simulink model "EPRModel_doublePulseStimulusCodeOffset"  (R2022a)
settings: Solver=ode5  StartTime=0.0  StopTime=inf  RelTol=1e-3
InitFcn:
  | eprecorder_mdl_init_callback();
StopFcn:
  | eprecorder_mdl_stop_callback;
undefined symbols (not defined in the file or in its folder): EPR, eprecorder_online_on_triggered, eprecorder_online_on_viewer_triggered
libraries: simulink x2, sldrtlib x1
settings Model: Creator=Neurolab  LastModifiedBy=bo11r
settings SolverCC: AlgebraicLoopSolver=TrustRegion
settings DebuggingCC: UnconnectedInputMsg=warning  UnconnectedOutputMsg=warning  UnconnectedLineMsg=warning  SFMachineParentedDataDiag=warning
settings RTWCC: Description=Simulink Desktop Real-Time  SystemTargetFile=sldrt.tlc  TemplateMakefile=sldrt.tmf  RTWCompilerOptimization=on  DLArmComputeVersion=19.05
settings CodeAppCC: MaxIdLength=95
settings SimulinkDesktopRealTimeCC: TargetPreCompLibLocation=C:\Program Files\MATLAB\R2020b\toolbox\sldrt\lib\win64

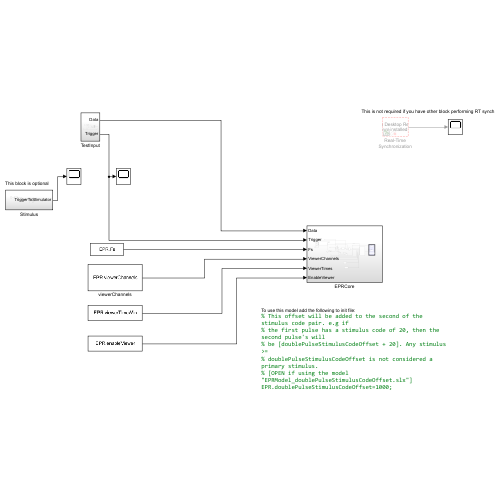
[thumbnail: Simulink's stored preview of the top-level diagram]
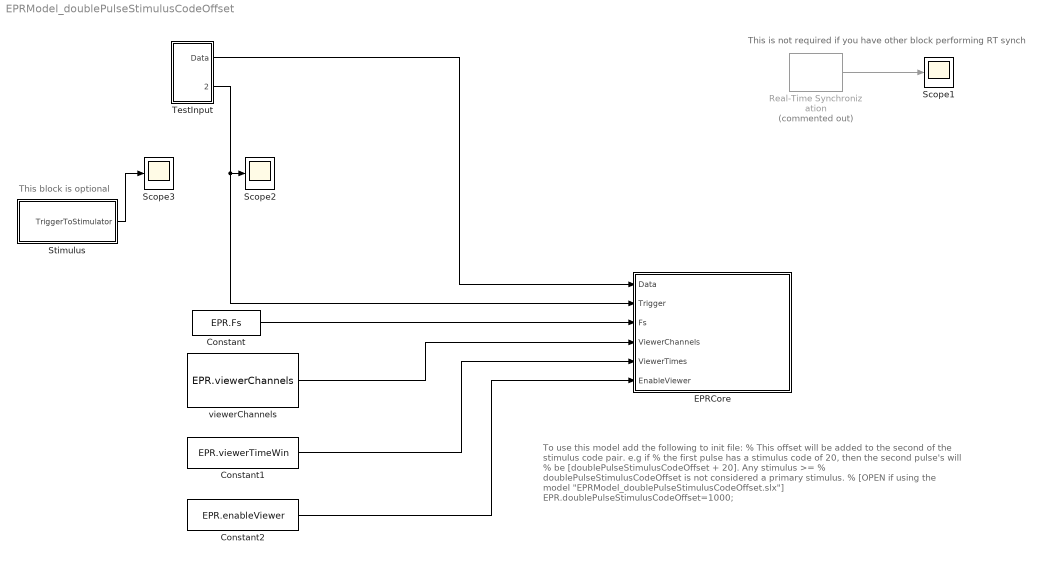
== system EPRModel_doublePulseStimulusCodeOffset ==
  note: To use this model add the following to init file:
      | % This offset will be added to the second of the stimulus code pair. e.g if
      | % the first pulse has a stimulus code of 20, then the second pulse's will
      | % be [doublePulseStimulusCodeOffset + 20]. Any stimulus >=
      | % doublePulseStimulusCodeOffset is not considered a primary stimulus.
      | % [OPEN if using the model "EPRModel_doublePulseStimulusCodeOffset.slx"]
      | EPR.doublePulseStimulusCodeOffset=1000;
  note: This block is optional
  note: This is not required if you have other block performing RT synch
  Constant : Constant  Value=EPR.Fs
  Constant1 : Constant  Value=EPR.viewerTimeWin
  Constant2 : Constant  Value=EPR.enableViewer
  EPRCore : Subsystem
  Real-Time Synchronization : sldrtlib/Real-Time Synchronization  Commented=on  SampleTime=1/EPR.Fs  MaxMissedTicks=1000  ShowMissedTicks=on  YieldWhenWaiting=off
  Scope1 : Scope
  Scope2 : Scope
  Scope3 : Scope
  Stimulus : Subsystem
  TestInput : Subsystem
  viewerChannels : Constant  Value=EPR.viewerChannels  mask(Creates axes for plottint EP){}
      mask init:
      | %{
      |  p=[403   246   560   420]
      |  u='pixels'
      | if(length(findobj('tag','EMG000')))
      |      h=figure(findobj('tag','EMG000'));
      |      p=get(h,'position');
      |      u=get(h,'units');
      |      close(h);
      | end
      |      figure1 = figure('numbertitle','off','name','EP','tag','EMG000');
      |      set(figure1,'units',u);
      |      set(figure1,'position',p);
      |      % Create axes
      |      MYEP.axes(1)=subplot(3,1,1);
      |       title('Channels 1 avg')
      |       box(MYEP.axes(1),'on');
      |       hold(MYEP.axes(1),'all');
      | 
      |      MYEP.axes(2)=subplot(3,1,2);
      |       title('Channels 2 avg')
      |       box(MYEP.axes(2),'on');
      |       hold(MYEP.axes(2),'all');
      | 
      |      MYEP.axes(3)=subplot(3,1,3);
      |      title('Channels 3 avg')
      |      xlabel('1 sec Samples since stimulus onset')
      |      ylabel('Avg amplitude (micro volts)')
      |      box(MYEP.axes(3),'on');
      |      hold(MYEP.axes(3),'all');
      | 
      | %}
  wires:
  viewerChannels/1 -> EPRCore/4(ViewerChannels)
  Constant/1 -> EPRCore/3(Fs)
  Constant1/1 -> EPRCore/5(ViewerTimes)
  Constant2/1 -> EPRCore/6(EnableViewer)
  Real-Time Synchronization/1 -> Scope1/1
  TestInput/1(Data) -> EPRCore/1(Data)
  TestInput/2(Trigger) -> EPRCore/2(Trigger), Scope2/1
  Stimulus/1(TriggerToStimulator) -> Scope3/1

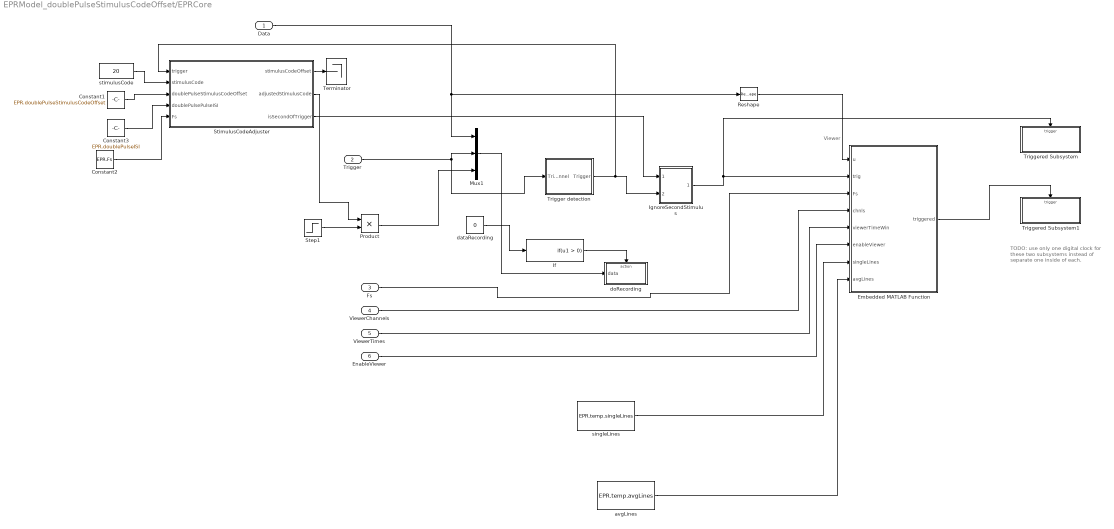
== system EPRModel_doublePulseStimulusCodeOffset/EPRCore ==
  note: TODO: use only one digital clock
      | for these two subsystems instead
      | of separate one inside of each.
  note: Viewer
  Data : Inport
  Trigger : Inport  Port=2
  Fs : Inport  Port=3
  ViewerChannels : Inport  Port=4
  ViewerTimes : Inport  Port=5
  EnableViewer : Inport  Port=6
  Constant1 : Constant  Value=EPR.doublePulseStimulusCodeOffset
  Constant2 : Constant  Value=EPR.Fs
  Constant3 : Constant  Value=EPR.doublePulseISI
  Embedded MATLAB Function : MATLAB Function  TreatAsAtomicUnit=on
  If : If  ShowElse=off
  IgnoreSecondStimulus : Subsystem
  Mux1 : Mux  Inputs=3
  Product : Product
  Reshape : Reshape
  Step1 : Step  Before=1  SampleTime=0
  StimulusCodeAdjuster : MATLAB Function  TreatAsAtomicUnit=on
  Terminator : Terminator
  Trigger detection : Subsystem
  Triggered Subsystem : Subsystem  TreatAsAtomicUnit=on
  Triggered Subsystem1 : Subsystem  TreatAsAtomicUnit=on
  avgLines : Constant  Value=EPR.temp.avgLines  mask(Creates axes for plottint EP){}
      mask init: same as EPRModel_doublePulseStimulusCodeOffset/viewerChannels
  dataRecording : Constant  Value=0
  doRecording : Subsystem  TreatAsAtomicUnit=on
  singleLines : Constant  Value=EPR.temp.singleLines  mask(Creates axes for plottint EP){}
      mask init: same as EPRModel_doublePulseStimulusCodeOffset/viewerChannels
  stimulusCode : Constant  Value=20
  wires:
  If/1 -> doRecording/Action
  Data/1 -> Mux1/1, Reshape/1
  dataRecording/1 -> If/1
  ViewerChannels/1 -> Embedded MATLAB Function/4(chnls)
  Trigger/1 -> Mux1/2, Trigger detection/1(Trigger channel)
  Mux1/1 -> doRecording/1(data)
  Fs/1 -> Embedded MATLAB Function/3(Fs)
  ViewerTimes/1 -> Embedded MATLAB Function/5(viewerTimeWin)
  EnableViewer/1 -> Embedded MATLAB Function/6(enableViewer)
  Reshape/1 -> Embedded MATLAB Function/1(u)
  Step1/1 -> Product/2
  Product/1 -> Mux1/3
  singleLines/1 -> Embedded MATLAB Function/7(singleLines)
  avgLines/1 -> Embedded MATLAB Function/8(avgLines)
  Embedded MATLAB Function/1(triggered) -> Triggered Subsystem1/Trigger
  IgnoreSecondStimulus/1(Trigger) -> Triggered Subsystem/Trigger, Embedded MATLAB Function/2(trig)
  Trigger detection/1(Trigger) -> StimulusCodeAdjuster/1(trigger), IgnoreSecondStimulus/2(TriggerIn)
  StimulusCodeAdjuster/3(isSecondOfTrigger) -> IgnoreSecondStimulus/1(isSecondTrigger)
  stimulusCode/1 -> StimulusCodeAdjuster/2(stimulusCode)
  Constant1/1 -> StimulusCodeAdjuster/3(doublePulseStimulusCodeOffset)
  Constant2/1 -> StimulusCodeAdjuster/5(Fs)
  Constant3/1 -> StimulusCodeAdjuster/4(doublePulsePulseISI)
  StimulusCodeAdjuster/2(adjustedStimulusCode) -> Product/1
  StimulusCodeAdjuster/1(stimulusCodeOffset) -> Terminator/1

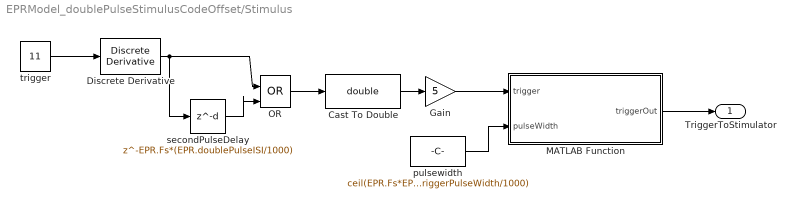
== system EPRModel_doublePulseStimulusCodeOffset/Stimulus ==
  Cast To Double : DataTypeConversion  OutDataTypeStr=double  SaturateOnIntegerOverflow=off  RndMeth=Floor
  Discrete Derivative : simulink/Discrete/Discrete Derivative  gainval=1.0  ICPrevScaledInput=0.0  OutMin=[]  OutMax=[]  OutDataType=fixdt(1, 16)  OutScaling=2^-10  DoSatur=off
  Gain : Gain  Gain=5
  MATLAB Function : MATLAB Function  TreatAsAtomicUnit=on
  OR : Logic  Operator=OR  IconShape=distinctive  AllPortsSameDT=off  OutDataTypeStr=boolean
  pulsewidth : Constant  Value=ceil(EPR.Fs*EPR.stimulusTriggerPulseWidth/1000)
  secondPulseDelay : Delay  DelayLength=EPR.Fs*(EPR.doublePulseISI/1000)
  trigger : Constant  Value=11
  TriggerToStimulator : Outport
  wires:
  secondPulseDelay/1 -> OR/2
  OR/1 -> Cast To Double/1
  trigger/1 -> Discrete Derivative/1
  Discrete Derivative/1 -> secondPulseDelay/1, OR/1
  Cast To Double/1 -> Gain/1
  Gain/1 -> MATLAB Function/1(trigger)
  pulsewidth/1 -> MATLAB Function/2(pulseWidth)
  MATLAB Function/1(triggerOut) -> TriggerToStimulator/1

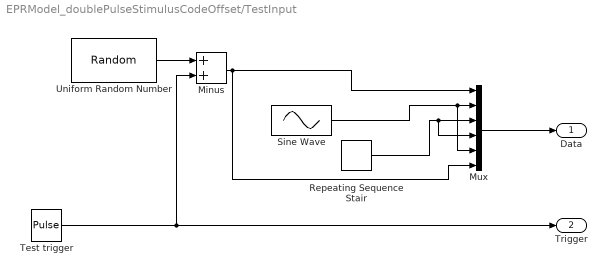
== system EPRModel_doublePulseStimulusCodeOffset/TestInput ==
  Minus : Sum
  Mux : Mux  Inputs=6
  Repeating Sequence Stair : simulink/Sources/Repeating Sequence Stair  OutValues=[3 1 4 2 1].'  tsamp=-1  OutMin=[]  OutMax=[]  OutDataTypeStr=double  OutputDataTypeScalingMode=double  OutDataType=fixdt(0,8)  ConRadixGroup=Best Precision: Vector-wise  OutScaling=2^-12
  Sine Wave : Sin  SampleTime=0
  Test trigger : DiscretePulseGenerator  Amplitude=4  Period=3*EPR.Fs  PulseWidth=max(round(0.001*EPR.Fs),1)  SampleTime=1/EPR.Fs
  Uniform Random Number : UniformRandomNumber  SampleTime=1/EPR.Fs
  Data : Outport
  Trigger : Outport  Port=2
  wires:
  Mux/1 -> Data/1
  Uniform Random Number/1 -> Minus/1
  Repeating Sequence Stair/1 -> Mux/4, Mux/3
  Sine Wave/1 -> Mux/5, Mux/2
  Test trigger/1 -> Minus/2, Trigger/1
  Minus/1 -> Mux/6, Mux/1

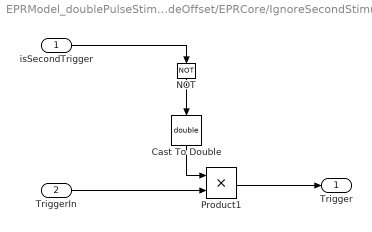
== system EPRModel_doublePulseStimulusCodeOffset/EPRCore/IgnoreSecondStimulus ==
  isSecondTrigger : Inport
  TriggerIn : Inport  Port=2
  Cast To Double : DataTypeConversion  OutDataTypeStr=double  SaturateOnIntegerOverflow=off  RndMeth=Floor
  NOT : Logic  Operator=NOT  IconShape=distinctive  AllPortsSameDT=off  OutDataTypeStr=boolean
  Product1 : Product
  Trigger : Outport
  wires:
  isSecondTrigger/1 -> NOT/1
  TriggerIn/1 -> Product1/2
  Cast To Double/1 -> Product1/1
  Product1/1 -> Trigger/1
  NOT/1 -> Cast To Double/1

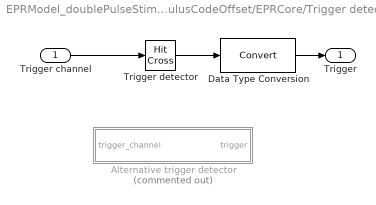
== system EPRModel_doublePulseStimulusCodeOffset/EPRCore/Trigger detection ==
  Trigger channel : Inport
  Alternative trigger detector : MATLAB Function  Commented=on  TreatAsAtomicUnit=on
  Data Type Conversion : DataTypeConversion  SaturateOnIntegerOverflow=off  RndMeth=Floor
  Trigger detector : HitCross  HitCrossingOffset=1  HitCrossingDirection=rising
  Trigger : Outport
  wires:
  Trigger detector/1 -> Data Type Conversion/1
  Trigger channel/1 -> Trigger detector/1
  Data Type Conversion/1 -> Trigger/1

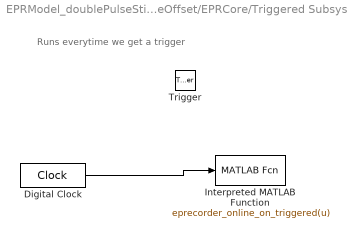
== system EPRModel_doublePulseStimulusCodeOffset/EPRCore/Triggered Subsystem ==
  note: Runs everytime we get a trigger
  Trigger : TriggerPort  TriggerTime=on sample time hit  VariantControl=(inherit)
  Digital Clock : DigitalClock  SampleTime=-1
  Interpreted MATLAB Function : MATLABFcn  MATLABFcn=eprecorder_online_on_triggered(u)  OutputDimensions=0
  wires:
  Digital Clock/1 -> Interpreted MATLAB Function/1

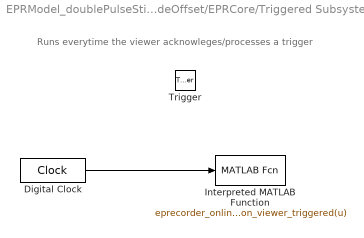
== system EPRModel_doublePulseStimulusCodeOffset/EPRCore/Triggered Subsystem1 ==
  note: Runs everytime the viewer acknowleges/processes a trigger
  Trigger : TriggerPort  TriggerTime=on sample time hit  VariantControl=(inherit)
  Digital Clock : DigitalClock  SampleTime=-1
  Interpreted MATLAB Function : MATLABFcn  MATLABFcn=eprecorder_online_on_viewer_triggered(u)  OutputDimensions=0
  wires:
  Digital Clock/1 -> Interpreted MATLAB Function/1

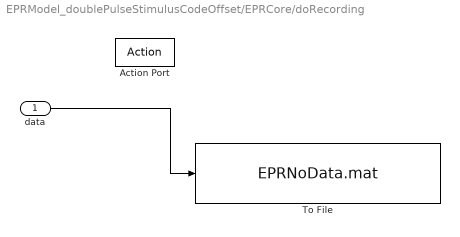
== system EPRModel_doublePulseStimulusCodeOffset/EPRCore/doRecording ==
  data : Inport
  Action Port : ActionPort  ActionPortLabel=if(u1 > 0)
  To File : ToFile  Filename=EPRNoData.mat  MatrixName=EPdata
  wires:
  data/1 -> To File/1

== matlab function EPRModel_doublePulseStimulusCodeOffset/EPRCore/Embedded MATLAB Function ==
  data: u input; trig input; Fs input; chnls input; viewerTimeWin input; enableViewer input; singleLines input; avgLines input; triggered output
function triggered=fcn(u,trig,Fs,chnls,viewerTimeWin,enableViewer,singleLines,avgLines)
%#codegen
coder.extrinsic('set');
%% EPR viewer
% [INPUT]
% u: Current data.
% trig: Trigger channel. Trigger is detected when value is 1 or greater. A
% trigger is ignored if it collides with a previous trigger. The implicit
% collision detection is based on viewerTimeWin arguement.
% Fs: Sample rate.
% chnls: the indexes of channels to display.
% viewerTimeWin: Two element vector. Where the first element is the start time
%   and the second element is end time in ms for window of data to display. 
% enableViewer: When equivalent to false, nothing will be done.
% singleLines: The main data line plot handles for each axes for non-avg
%   data where latest data will be plotted. Must correspond to chnls.
% avgAxes: The line plot handles where to display the running avg. Must
%   correspond to chnls.
% [OUTPUT]
% triggered: int<0,1> A value of 1 if trigger recieved is acknowledged or
%   processed and value of zero no trigger is recieved or trigger sent is
%   ignored because it collided with a previous trigger.
% 
persistent bufferData sumData sT numAVG tAxes recordLen;

triggered=0;

if(~enableViewer)
    return
end

if(isempty(bufferData))% init
    
    sT=-1;
    numAVG=0;%increamented at each trigger to count the number of averages
    
    % Display window sample samples
    dispWin=zeros(2,1);
    dispWin(1)=round(viewerTimeWin(1)/1000*Fs) +1;% convert to sample. We add 1 b/c matlab starts at 1 but time starts at zero
    dispWin(2)=round(viewerTimeWin(2)/1000*Fs) +1;% convert to smaple.
    tAxes=(dispWin(1)-1:dispWin(2)-1)/Fs*1000;% We subtract 1 b/c samples in matlab starts from 1 while time start from zero.
    
    % Data Buffer
    recordLen=dispWin(2); %i.e the length of data to acquire start from trigger to the end
    
    bufferLen=dispWin(2)-dispWin(1)+1;% we add 1 because to make it inclusive of the starting point, i.e dispWin(1). We can also get this as length(tAxes).
    
    % Data
    nChnls=length(chnls);%number of channels
    sumData=zeros(bufferLen,nChnls);

    bufferData=zeros(bufferLen,nChnls);
    
end

% Fifo. Append new data at the end
bufferData(1:end-1,:)=bufferData(2:end,:);
bufferData(end,:)=u(chnls)';


%collect data only at onset of stimulation if 'sT'<0 ('sT'<0 =>avoid
%collision of triggers by ignoring subsequent triggers untill 'data1' is
%filled. Actually it is better to allow the trigger to restart if trigers
%collide but this will lead to wrong number of averages. The best solution
%is not to let triggers collide. One trigger period is the onset of the
%trigger to the time the data for the trigger is collected)     
if trig(1) >=1 && sT<0 
    sT=recordLen;
    triggered=1;
end
sT=sT-1;


if sT==0
   
   sumData=sumData+bufferData;
   numAVG=numAVG+1;

   for n=1:length(chnls)
       
       %Plot last window
       if(numAVG==1)% The x-axes only need to be set once
           set(singleLines(n),'XData',tAxes);
       end
       set(singleLines(n),'YData',bufferData(:,n));
       
       
       % Plo avg
       if(numAVG==1)% The x-axes only need to be set once
           set(avgLines(n),'XData',tAxes);
       end
       set(avgLines(n),'YData',sumData(:,n)/numAVG);
   end
    
end
% all that glitter is not gold;http://www.youtube.com/watch?v=LWK4NWS479s

== matlab function EPRModel_doublePulseStimulusCodeOffset/EPRCore/Trigger detection/Alternative trigger detector ==
  data: trigger_channel input; trigger output
function trigger = fcn(trigger_channel)
% Outputs 1 when trigger_channel is at least 1, or zero otherwise.
persistent prev_trigger_channel;

thresh=1;% detection threshold

if(isempty(prev_trigger_channel))
    prev_trigger_channel=0;
end

trigger=0;
if( (trigger_channel-prev_trigger_channel) >=thresh)
    trigger=1;
end

prev_trigger_channel=trigger_channel;

== matlab function EPRModel_doublePulseStimulusCodeOffset/EPRCore/StimulusCodeAdjuster ==
  data: stimulusCodeOffset output; trigger input; adjustedStimulusCode output; stimulusCode input; doublePulseStimulusCodeOffset input; doublePulsePulseISI input; Fs input; isSecondOfTrigger output
function [stimulusCodeOffset,adjustedStimulusCode,isSecondOfTrigger]  = fcn(trigger,stimulusCode,doublePulseStimulusCodeOffset,doublePulsePulseISI,Fs)
% Adjust the stimulus code after detecting the second stimulus pair.
%
% trigger:{0,1} 1=>trigger detected.
% stimulusCode: The currebt stimulus code.
% doublePulseStimulusCodeOffset: The code used to offset the second of the
%   double paired stimuli. 
% doublePulsePulseISI: Inter stimulus interval.
% Fs: Samplerate
%
% stimulusCodeOffset: The offset to be used to adjust stimulus code.
% adjustedStimulusCode: The adjusted stimulus code.  
% isSecondOfTrigger: {0,1} 1 =>the current trigger is the second of the
%   double pair.
%
persistent t;
if(isempty(t))
    t=-1;
end


isSecondOfTrigger=0;

if(trigger && t==-1)% detect first of pair
    t=doublePulsePulseISI*Fs/1000;
end

if(trigger && t==0) % detect second of pair. TODO:WHAT IF trigger DOES NOT OCCURE AT EXACTLY ZERO.
    stimulusCodeOffset=doublePulseStimulusCodeOffset;
    t=-1;
    isSecondOfTrigger=1;
end

if(t>-1)
    t=t-1;
end

adjustedStimulusCode=stimulusCode+stimulusCodeOffset;

== matlab function EPRModel_doublePulseStimulusCodeOffset/Stimulus/MATLAB Function ==
  data: trigger input; triggerOut output; pulseWidth input
function triggerOut = fcn(trigger,pulseWidth)
    % Hold the trigger until pulse width is reached.
    % [INPUT]
    % trigger: the value of the trigger.
    % pulseWidth: the pulse width in samples.

    persistent heldTrigger t;
    if isempty(t)
        t=0;
        heldTrigger=0;
    end

    if trigger>0
        t=pulseWidth;
        heldTrigger=trigger;
    end
    
    if(t>0)
        t=t-1;
        triggerOut=heldTrigger;
    else
        triggerOut=trigger;
    end
